simulink library "maggyroProcessing_lib"  (R2018b)
settings: Solver=VariableStepAuto  StartTime=0.0  StopTime=10.0  RelTol=1e-3
undefined symbols (not defined in the file or in its folder): fswParams, u1, unit_conversion
libraries: dspindex x18, two_norm x9, simulink x7
settings Model: Creator=sophiakim  LastModifiedBy=Taylor

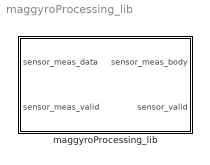
== system maggyroProcessing_lib ==
  maggyroProcessing_lib : Subsystem  TreatAsAtomicUnit=on  mask{static_range_max_value=fswParams.sensors.gyro_static_range, offset_calibration_matrix=fswParams.sensors.gyro_offset, max_err=fswParams.sensors.mag_max_err, rotation_calibration_matrix=fswParams.sensors.gyro_rotate, Gain=unit_conversion}
      mask prompts: static_range_max_value "Max Static Range"; offset_calibration_matrix "Offset Calibration Matrix"; max_err "Max Error Between Signals Allowed"; rotation_calibration_matrix "3x3x3 Matrix of Rotation Matrices"; Gain "Measurement-to-FSW Unit Conversion"
      settings: RTWFcnNameOpts=Use subsystem name  RTWFileNameOpts=Use subsystem name
      mask TypeOptions static_range_max_value:
      | StaticRangeCheck
      | /Check
      | Static Range1/max | StaticRangeCheck
      | /Check
      | Static Range2/max | StaticRangeCheck
      | /Check
      | Static Range4/max
      mask TypeOptions offset_calibration_matrix: DataCalibration/mag_offset/Value
      mask TypeOptions Gain: UnitConversion/Gain
      mask DialogControl DescTextVar Prompt: Provide the sensor (mag or gyro) measurements in the sensor frame(s), as well as the individual validity flags. This library then blends the three measurements into a single three-dimensional vector and a single validity flag.

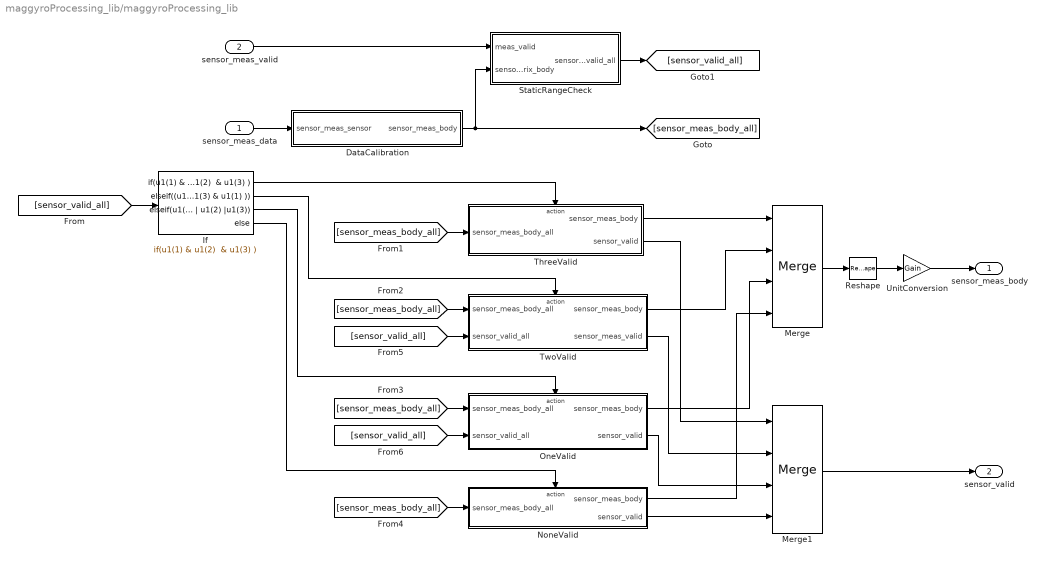
== system maggyroProcessing_lib/maggyroProcessing_lib ==
  sensor_meas_data : Inport
  sensor_meas_valid : Inport  Port=2
  DataCalibration : Subsystem
  If : If  IfExpression="u1(1) & u1(2)  & u1(3)"  ElseIfExpressions=(u1(1) & u1(2) ) | (u1(2) & u1(3) )|(u1(3) & u1(1) ), u1(1) | u1(2) |u1(3)
  Merge : Merge  Inputs=4
  Merge1 : Merge  Inputs=4
  NoneValid : Subsystem  TreatAsAtomicUnit=on
  OneValid : Subsystem  TreatAsAtomicUnit=on
  Reshape : Reshape
  "StaticRangeCheck " : Subsystem
  ThreeValid : Subsystem  TreatAsAtomicUnit=on
  TwoValid : Subsystem  TreatAsAtomicUnit=on
  UnitConversion : Gain  Gain=Gain
  sensor_meas_body : Outport
  sensor_valid : Outport  Port=2
  wires:
  "StaticRangeCheck "/1(sensor_valid_all) -> [sensor_valid_all]
  NoneValid/2(sensor_valid) -> Merge1/4
  If/4 -> NoneValid/Action
  [sensor_valid_all] -> If/1
  [sensor_meas_body_all] -> OneValid/1(sensor_meas_body_all)
  [sensor_valid_all] -> OneValid/2(sensor_valid_all)
  OneValid/1(sensor_meas_body) -> Merge/3
  TwoValid/2(sensor_meas_valid) -> Merge1/2
  NoneValid/1(sensor_meas_body) -> Merge/4
  [sensor_meas_body_all] -> TwoValid/1(sensor_meas_body_all)
  If/1 -> ThreeValid/Action
  If/2 -> TwoValid/Action
  If/3 -> OneValid/Action
  OneValid/2(sensor_valid) -> Merge1/3
  TwoValid/1(sensor_meas_body) -> Merge/2
  [sensor_meas_body_all] -> NoneValid/1(sensor_meas_body_all)
  [sensor_valid_all] -> TwoValid/2(sensor_valid_all)
  Merge/1 -> Reshape/1
  Merge1/1 -> sensor_valid/1
  sensor_meas_valid/1 -> "StaticRangeCheck "/1(meas_valid)
  sensor_meas_data/1 -> DataCalibration/1(sensor_meas_sensor)
  DataCalibration/1(sensor_meas_body) -> "StaticRangeCheck "/2(sensor_matrix_body), [sensor_meas_body_all]
  ThreeValid/1(sensor_meas_body) -> Merge/1
  ThreeValid/2(sensor_valid) -> Merge1/1
  [sensor_meas_body_all] -> ThreeValid/1(sensor_meas_body_all)
  Reshape/1 -> UnitConversion/1
  UnitConversion/1 -> sensor_meas_body/1

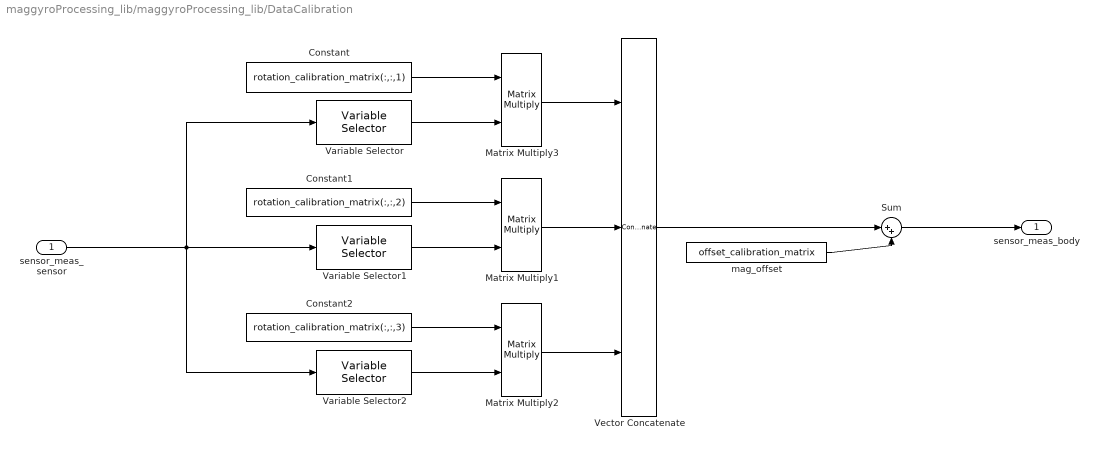
== system maggyroProcessing_lib/maggyroProcessing_lib/DataCalibration ==
  sensor_meas_sensor : Inport
  Constant : Constant  Value=rotation_calibration_matrix(:,:,1)
  Constant1 : Constant  Value=rotation_calibration_matrix(:,:,2)
  Constant2 : Constant  Value=rotation_calibration_matrix(:,:,3)
  Matrix Multiply1 : Product  Multiplication=Matrix(*)
  Matrix Multiply2 : Product  Multiplication=Matrix(*)
  Matrix Multiply3 : Product  Multiplication=Matrix(*)
  Sum : Sum  Inputs=|++
  Variable Selector : dspindex/Variable Selector  NumInputs=1  rowsOrCols=Columns  IdxMode=Fixed  Elements=[1]  ZerOneIdxMode=One-based  errmode=Clip Index  FillMode=on  FillValues=0
  Variable Selector1 : dspindex/Variable Selector  NumInputs=1  rowsOrCols=Columns  IdxMode=Fixed  Elements=[2]  ZerOneIdxMode=One-based  errmode=Clip Index  FillMode=on  FillValues=0
  Variable Selector2 : dspindex/Variable Selector  NumInputs=1  rowsOrCols=Columns  IdxMode=Fixed  Elements=[3]  ZerOneIdxMode=One-based  errmode=Clip Index  FillMode=on  FillValues=0
  Vector Concatenate : Concatenate  NumInputs=3  Mode=Multidimensional array  ConcatenateDimension=2
  mag_offset : Constant  Value=offset_calibration_matrix
  sensor_meas_body : Outport
  wires:
  mag_offset/1 -> Sum/2
  Sum/1 -> sensor_meas_body/1
  sensor_meas_sensor/1 -> Variable Selector/1, Variable Selector2/1, Variable Selector1/1
  Variable Selector/1 -> Matrix Multiply3/2
  Constant/1 -> Matrix Multiply3/1
  Variable Selector1/1 -> Matrix Multiply1/2
  Variable Selector2/1 -> Matrix Multiply2/2
  Constant1/1 -> Matrix Multiply1/1
  Constant2/1 -> Matrix Multiply2/1
  Matrix Multiply3/1 -> Vector Concatenate/1
  Matrix Multiply1/1 -> Vector Concatenate/2
  Matrix Multiply2/1 -> Vector Concatenate/3
  Vector Concatenate/1 -> Sum/1

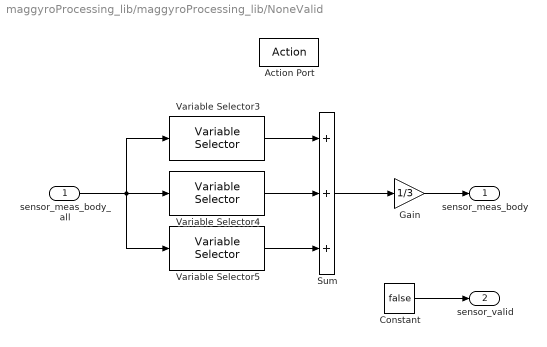
== system maggyroProcessing_lib/maggyroProcessing_lib/NoneValid ==
  sensor_meas_body_all : Inport
  Action Port : ActionPort
  Constant : Constant  Value=false
  Gain : Gain  Gain=1/3
  Sum : Sum  Inputs=+++
  Variable Selector3 : dspindex/Variable Selector  NumInputs=1  rowsOrCols=Columns  IdxMode=Fixed  Elements=[1]  ZerOneIdxMode=One-based  errmode=Clip Index  FillMode=on  FillValues=0
  Variable Selector4 : dspindex/Variable Selector  NumInputs=1  rowsOrCols=Columns  IdxMode=Fixed  Elements=[2]  ZerOneIdxMode=One-based  errmode=Clip Index  FillMode=on  FillValues=0
  Variable Selector5 : dspindex/Variable Selector  NumInputs=1  rowsOrCols=Columns  IdxMode=Fixed  Elements=[3]  ZerOneIdxMode=One-based  errmode=Clip Index  FillMode=on  FillValues=0
  sensor_meas_body : Outport
  sensor_valid : Outport  Port=2
  wires:
  Sum/1 -> Gain/1
  Variable Selector5/1 -> Sum/3
  Variable Selector4/1 -> Sum/2
  Variable Selector3/1 -> Sum/1
  sensor_meas_body_all/1 -> Variable Selector5/1, Variable Selector3/1, Variable Selector4/1
  Gain/1 -> sensor_meas_body/1
  Constant/1 -> sensor_valid/1

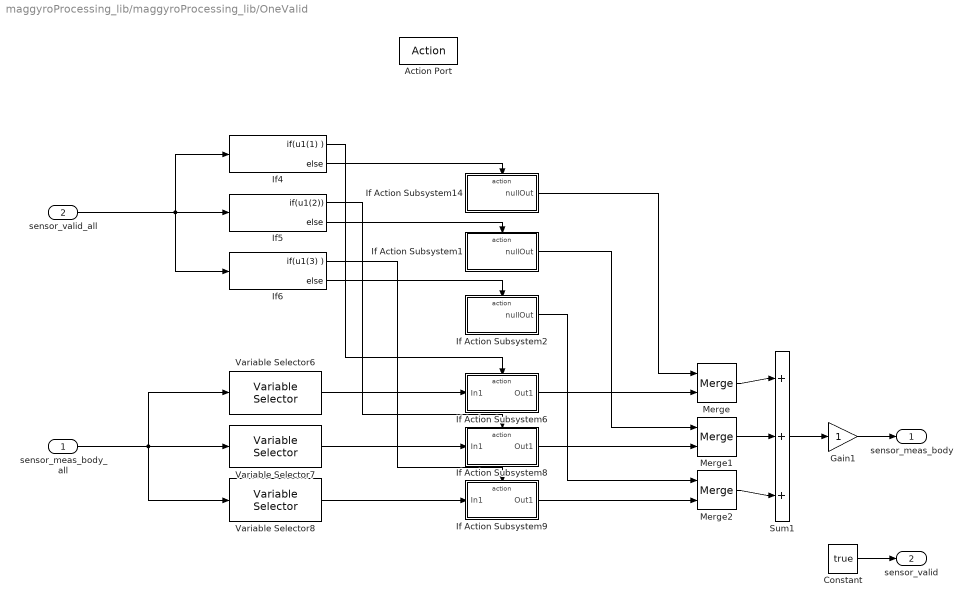
== system maggyroProcessing_lib/maggyroProcessing_lib/OneValid ==
  sensor_meas_body_all : Inport
  sensor_valid_all : Inport  Port=2
  Action Port : ActionPort
  Constant : Constant  Value=true
  Gain1 : Gain
  If Action Subsystem1 : Subsystem  TreatAsAtomicUnit=on
  If Action Subsystem14 : Subsystem  TreatAsAtomicUnit=on
  If Action Subsystem2 : Subsystem  TreatAsAtomicUnit=on
  If Action Subsystem6 : Subsystem  TreatAsAtomicUnit=on
  If Action Subsystem8 : Subsystem  TreatAsAtomicUnit=on
  If Action Subsystem9 : Subsystem  TreatAsAtomicUnit=on
  If4 : If  IfExpression=u1(1)
  If5 : If  IfExpression=u1(2)
  If6 : If  IfExpression=u1(3)
  Merge : Merge
  Merge1 : Merge
  Merge2 : Merge
  Sum1 : Sum  Inputs=+++
  Variable Selector6 : dspindex/Variable Selector  NumInputs=1  rowsOrCols=Columns  IdxMode=Fixed  Elements=[1]  ZerOneIdxMode=One-based  errmode=Clip Index  FillMode=on  FillValues=0
  Variable Selector7 : dspindex/Variable Selector  NumInputs=1  rowsOrCols=Columns  IdxMode=Fixed  Elements=[2]  ZerOneIdxMode=One-based  errmode=Clip Index  FillMode=on  FillValues=0
  Variable Selector8 : dspindex/Variable Selector  NumInputs=1  rowsOrCols=Columns  IdxMode=Fixed  Elements=[3]  ZerOneIdxMode=One-based  errmode=Clip Index  FillMode=on  FillValues=0
  sensor_meas_body : Outport
  sensor_valid : Outport  Port=2
  wires:
  Gain1/1 -> sensor_meas_body/1
  If Action Subsystem6/1(Out1) -> Merge/2
  If4/2 -> If Action Subsystem14/Action
  If6/1 -> If Action Subsystem9/Action
  Sum1/1 -> Gain1/1
  If4/1 -> If Action Subsystem6/Action
  Variable Selector8/1 -> If Action Subsystem9/1(In1)
  Variable Selector6/1 -> If Action Subsystem6/1(In1)
  If Action Subsystem1/1(nullOut) -> Merge1/1
  If5/1 -> If Action Subsystem8/Action
  Merge/1 -> Sum1/1
  If Action Subsystem9/1(Out1) -> Merge2/2
  If Action Subsystem2/1(nullOut) -> Merge2/1
  Merge2/1 -> Sum1/3
  If Action Subsystem8/1(Out1) -> Merge1/2
  Variable Selector7/1 -> If Action Subsystem8/1(In1)
  Merge1/1 -> Sum1/2
  If6/2 -> If Action Subsystem2/Action
  If Action Subsystem14/1(nullOut) -> Merge/1
  If5/2 -> If Action Subsystem1/Action
  sensor_meas_body_all/1 -> Variable Selector6/1, Variable Selector8/1, Variable Selector7/1
  sensor_valid_all/1 -> If6/1, If4/1, If5/1
  Constant/1 -> sensor_valid/1

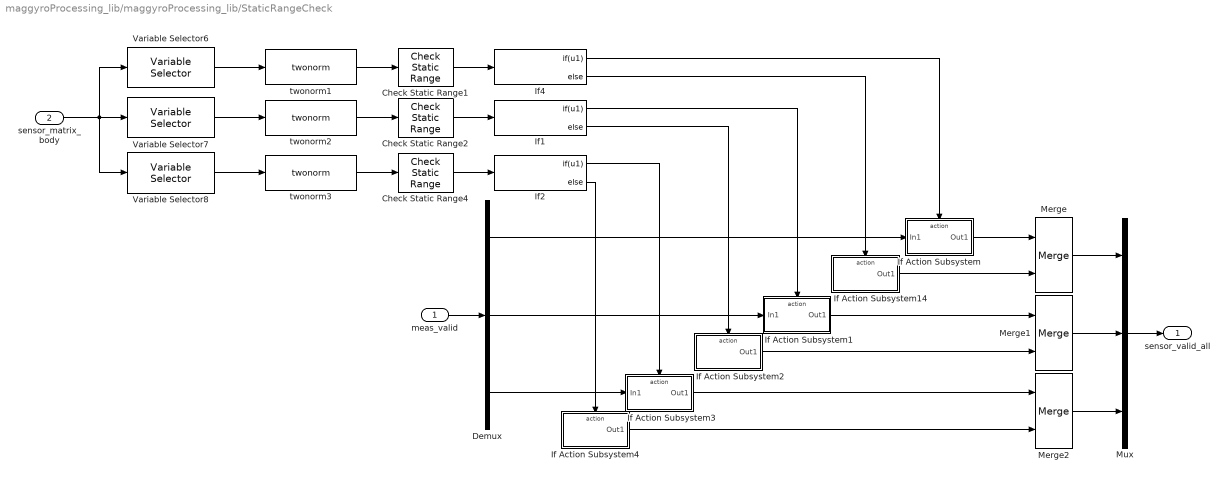
== system maggyroProcessing_lib/maggyroProcessing_lib/StaticRangeCheck  ==
  meas_valid : Inport
  sensor_matrix_body : Inport  Port=2
  Check Static Range1 : simulink/Model Verification/Check  Static Range  Description=0 <= u <= static_range_max_value  max=static_range_max_value  max_included=on  min=0  min_included=on  enabled=on  stopWhenAssertionFail=off  export=on  icon=graphic
      settings: SourceProductName=Simulink  SourceProductBaseCode=SL
  Check Static Range2 : simulink/Model Verification/Check  Static Range  Description=0 <= u <= static_range_max_value  max=static_range_max_value  max_included=on  min=0  min_included=on  enabled=on  stopWhenAssertionFail=off  export=on  icon=graphic
      settings: SourceProductName=Simulink  SourceProductBaseCode=SL
  Check Static Range4 : simulink/Model Verification/Check  Static Range  Description=0 <= u <= static_range_max_value  max=static_range_max_value  max_included=on  min=0  min_included=on  enabled=on  stopWhenAssertionFail=off  export=on  icon=graphic
      settings: SourceProductName=Simulink  SourceProductBaseCode=SL
  Demux : Demux  Outputs=3
  If Action Subsystem : Subsystem  TreatAsAtomicUnit=on
  If Action Subsystem1 : Subsystem  TreatAsAtomicUnit=on
  If Action Subsystem14 : Subsystem  TreatAsAtomicUnit=on
  If Action Subsystem2 : Subsystem  TreatAsAtomicUnit=on
  If Action Subsystem3 : Subsystem  TreatAsAtomicUnit=on
  If Action Subsystem4 : Subsystem  TreatAsAtomicUnit=on
  If1 : If  IfExpression=u1
  If2 : If  IfExpression=u1
  If4 : If  IfExpression=u1
  Merge : Merge
  Merge1 : Merge
  Merge2 : Merge
  Mux : Mux  Inputs=3
  Variable Selector6 : dspindex/Variable Selector  NumInputs=1  rowsOrCols=Columns  IdxMode=Fixed  Elements=[1]  ZerOneIdxMode=One-based  errmode=Clip Index  FillMode=on  FillValues=0
  Variable Selector7 : dspindex/Variable Selector  NumInputs=1  rowsOrCols=Columns  IdxMode=Fixed  Elements=[2]  ZerOneIdxMode=One-based  errmode=Clip Index  FillMode=on  FillValues=0
  Variable Selector8 : dspindex/Variable Selector  NumInputs=1  rowsOrCols=Columns  IdxMode=Fixed  Elements=[3]  ZerOneIdxMode=One-based  errmode=Clip Index  FillMode=on  FillValues=0
  twonorm1 : two_norm/twonorm  SystemSampleTime=-1
  twonorm2 : two_norm/twonorm  SystemSampleTime=-1
  twonorm3 : two_norm/twonorm  SystemSampleTime=-1
  sensor_valid_all : Outport
  wires:
  If2/2 -> If Action Subsystem4/Action
  If2/1 -> If Action Subsystem3/Action
  If4/2 -> If Action Subsystem14/Action
  Check Static Range1/1 -> If4/1
  If4/1 -> If Action Subsystem/Action
  Check Static Range4/1 -> If2/1
  If1/2 -> If Action Subsystem2/Action
  Demux/1 -> If Action Subsystem/1(In1)
  If1/1 -> If Action Subsystem1/Action
  If Action Subsystem/1(Out1) -> Merge/1
  If Action Subsystem14/1(Out1) -> Merge/2
  If Action Subsystem1/1(Out1) -> Merge1/1
  If Action Subsystem2/1(Out1) -> Merge1/2
  If Action Subsystem3/1(Out1) -> Merge2/1
  If Action Subsystem4/1(Out1) -> Merge2/2
  Demux/3 -> If Action Subsystem3/1(In1)
  Merge/1 -> Mux/1
  Merge1/1 -> Mux/2
  Merge2/1 -> Mux/3
  Mux/1 -> sensor_valid_all/1
  sensor_matrix_body/1 -> Variable Selector8/1, Variable Selector7/1, Variable Selector6/1
  Check Static Range2/1 -> If1/1
  Variable Selector6/1 -> twonorm1/1
  Variable Selector7/1 -> twonorm2/1
  Variable Selector8/1 -> twonorm3/1
  meas_valid/1 -> Demux/1
  Demux/2 -> If Action Subsystem1/1(In1)
  twonorm1/1 -> Check Static Range1/1
  twonorm2/1 -> Check Static Range2/1
  twonorm3/1 -> Check Static Range4/1

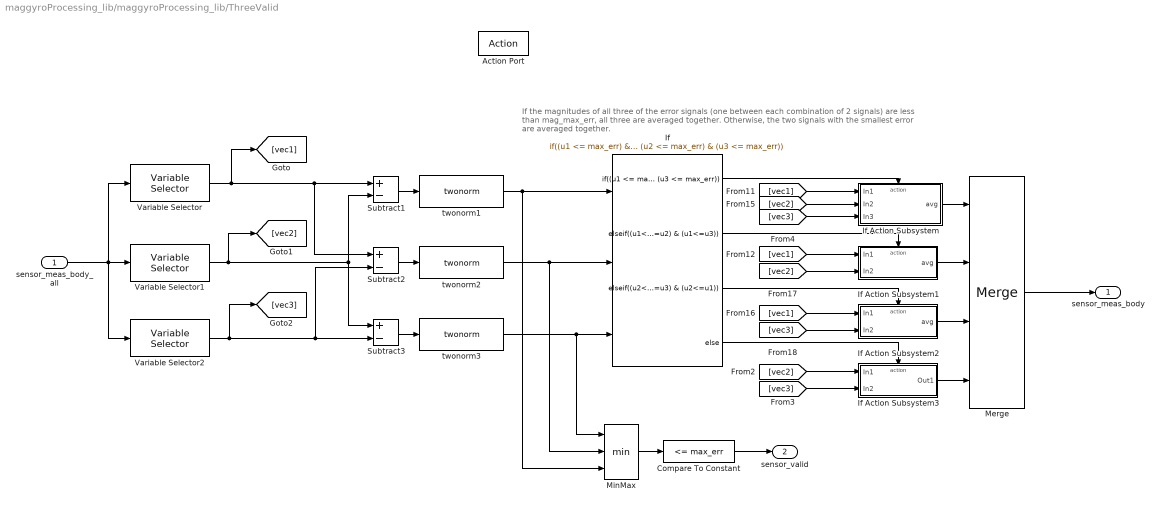
== system maggyroProcessing_lib/maggyroProcessing_lib/ThreeValid ==
  note: If the magnitudes of all three of the error signals (one between each combination of 2 signals)
      | are less than mag_max_err, all three are averaged together. Otherwise, the two signals with the
      | smallest error are averaged together.
  sensor_meas_body_all : Inport
  Action Port : ActionPort
  Compare To Constant : simulink/Logic and Bit Operations/Compare To Constant  relop=<=  const=max_err  OutDataTypeStr=boolean
  If : If  NumInputs=3  IfExpression=(u1 <= max_err) & (u2 <= max_err) & (u3 <= max_err)  ElseIfExpressions=(u1<=u2) & (u1<=u3),(u2<=u3) & (u2<=u1)
  If Action Subsystem : Subsystem  TreatAsAtomicUnit=on
  If Action Subsystem1 : Subsystem  TreatAsAtomicUnit=on
  If Action Subsystem2 : Subsystem  TreatAsAtomicUnit=on
  If Action Subsystem3 : Subsystem  TreatAsAtomicUnit=on
  Merge : Merge  Inputs=4
  MinMax : MinMax  Inputs=3
  Subtract1 : Sum  Inputs=+-
  Subtract2 : Sum  Inputs=+-
  Subtract3 : Sum  Inputs=+-
  Variable Selector : dspindex/Variable Selector  NumInputs=1  rowsOrCols=Columns  IdxMode=Fixed  Elements=[1]  ZerOneIdxMode=One-based  errmode=Clip Index  FillMode=on  FillValues=0
  Variable Selector1 : dspindex/Variable Selector  NumInputs=1  rowsOrCols=Columns  IdxMode=Fixed  Elements=[2]  ZerOneIdxMode=One-based  errmode=Clip Index  FillMode=on  FillValues=0
  Variable Selector2 : dspindex/Variable Selector  NumInputs=1  rowsOrCols=Columns  IdxMode=Fixed  Elements=[3]  ZerOneIdxMode=One-based  errmode=Clip Index  FillMode=on  FillValues=0
  twonorm1 : two_norm/twonorm  SystemSampleTime=-1
  twonorm2 : two_norm/twonorm  SystemSampleTime=-1
  twonorm3 : two_norm/twonorm  SystemSampleTime=-1
  sensor_meas_body : Outport
  sensor_valid : Outport  Port=2
  wires:
  twonorm3/1 -> MinMax/1, If/3
  twonorm2/1 -> MinMax/2, If/2
  twonorm1/1 -> MinMax/3, If/1
  Variable Selector/1 -> Subtract2/1, Subtract1/1, [vec1]
  Subtract1/1 -> twonorm1/1
  Subtract3/1 -> twonorm3/1
  [vec1] -> If Action Subsystem/1(In1)
  [vec1] -> If Action Subsystem1/1(In1)
  [vec2] -> If Action Subsystem/2(In2)
  [vec2] -> If Action Subsystem1/2(In2)
  Variable Selector1/1 -> Subtract1/2, Subtract3/1, [vec2]
  If/2 -> If Action Subsystem1/Action
  Variable Selector2/1 -> Subtract2/2, Subtract3/2, [vec3]
  If/3 -> If Action Subsystem2/Action
  Subtract2/1 -> twonorm2/1
  If/1 -> If Action Subsystem/Action
  If Action Subsystem/1(avg) -> Merge/1
  sensor_meas_body_all/1 -> Variable Selector/1, Variable Selector1/1, Variable Selector2/1
  If Action Subsystem1/1(avg) -> Merge/2
  If Action Subsystem2/1(avg) -> Merge/3
  Merge/1 -> sensor_meas_body/1
  MinMax/1 -> Compare To Constant/1
  Compare To Constant/1 -> sensor_valid/1
  [vec3] -> If Action Subsystem/3(In3)
  If/4 -> If Action Subsystem3/Action
  [vec3] -> If Action Subsystem2/2(In2)
  [vec1] -> If Action Subsystem2/1(In1)
  If Action Subsystem3/1(Out1) -> Merge/4
  [vec2] -> If Action Subsystem3/1(In1)
  [vec3] -> If Action Subsystem3/2(In2)

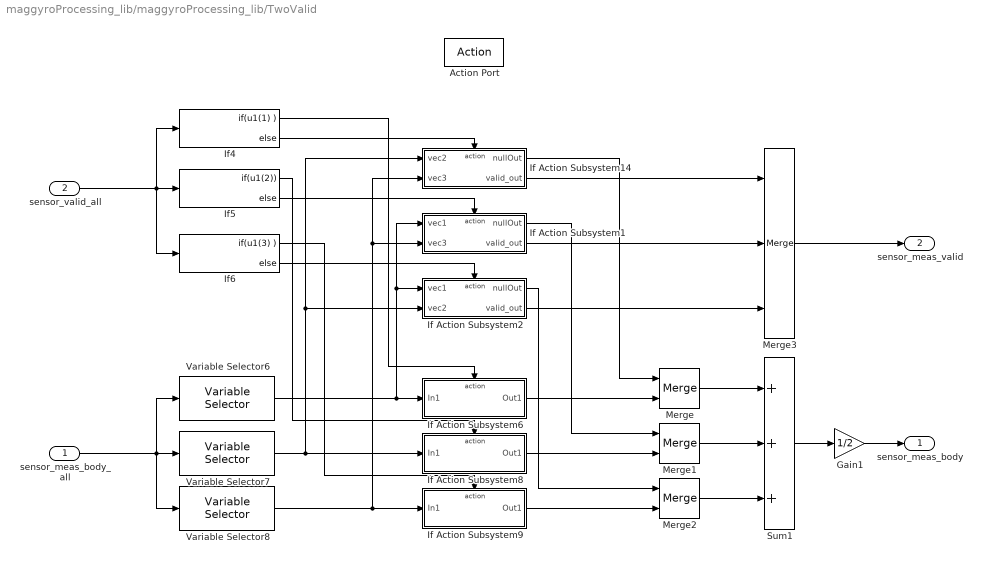
== system maggyroProcessing_lib/maggyroProcessing_lib/TwoValid ==
  sensor_meas_body_all : Inport
  sensor_valid_all : Inport  Port=2
  Action Port : ActionPort
  Gain1 : Gain  Gain=1/2
  If Action Subsystem1 : Subsystem  TreatAsAtomicUnit=on
  If Action Subsystem14 : Subsystem  TreatAsAtomicUnit=on
  If Action Subsystem2 : Subsystem  TreatAsAtomicUnit=on
  If Action Subsystem6 : Subsystem  TreatAsAtomicUnit=on
  If Action Subsystem8 : Subsystem  TreatAsAtomicUnit=on
  If Action Subsystem9 : Subsystem  TreatAsAtomicUnit=on
  If4 : If  IfExpression=u1(1)
  If5 : If  IfExpression=u1(2)
  If6 : If  IfExpression=u1(3)
  Merge : Merge
  Merge1 : Merge
  Merge2 : Merge
  Merge3 : Merge  Inputs=3
  Sum1 : Sum  Inputs=+++
  Variable Selector6 : dspindex/Variable Selector  NumInputs=1  rowsOrCols=Columns  IdxMode=Fixed  Elements=[1]  ZerOneIdxMode=One-based  errmode=Clip Index  FillMode=on  FillValues=0
  Variable Selector7 : dspindex/Variable Selector  NumInputs=1  rowsOrCols=Columns  IdxMode=Fixed  Elements=[2]  ZerOneIdxMode=One-based  errmode=Clip Index  FillMode=on  FillValues=0
  Variable Selector8 : dspindex/Variable Selector  NumInputs=1  rowsOrCols=Columns  IdxMode=Fixed  Elements=[3]  ZerOneIdxMode=One-based  errmode=Clip Index  FillMode=on  FillValues=0
  sensor_meas_body : Outport
  sensor_meas_valid : Outport  Port=2
  wires:
  Variable Selector7/1 -> If Action Subsystem2/2(vec2), If Action Subsystem14/1(vec2), If Action Subsystem8/1(In1)
  sensor_valid_all/1 -> If6/1, If4/1, If5/1
  If5/1 -> If Action Subsystem8/Action
  If6/1 -> If Action Subsystem9/Action
  If4/1 -> If Action Subsystem6/Action
  Variable Selector6/1 -> If Action Subsystem2/1(vec1), If Action Subsystem1/1(vec1), If Action Subsystem6/1(In1)
  Variable Selector8/1 -> If Action Subsystem1/2(vec3), If Action Subsystem14/2(vec3), If Action Subsystem9/1(In1)
  Gain1/1 -> sensor_meas_body/1
  Sum1/1 -> Gain1/1
  sensor_meas_body_all/1 -> Variable Selector8/1, Variable Selector7/1, Variable Selector6/1
  If4/2 -> If Action Subsystem14/Action
  If Action Subsystem14/1(nullOut) -> Merge/1
  If Action Subsystem6/1(Out1) -> Merge/2
  Merge/1 -> Sum1/1
  If Action Subsystem8/1(Out1) -> Merge1/2
  If Action Subsystem9/1(Out1) -> Merge2/2
  Merge2/1 -> Sum1/3
  Merge1/1 -> Sum1/2
  If5/2 -> If Action Subsystem1/Action
  If6/2 -> If Action Subsystem2/Action
  If Action Subsystem1/1(nullOut) -> Merge1/1
  If Action Subsystem2/1(nullOut) -> Merge2/1
  If Action Subsystem14/2(valid_out) -> Merge3/1
  If Action Subsystem1/2(valid_out) -> Merge3/2
  If Action Subsystem2/2(valid_out) -> Merge3/3
  Merge3/1 -> sensor_meas_valid/1

== system maggyroProcessing_lib/maggyroProcessing_lib/OneValid/If Action Subsystem1 ==
  Action Port : ActionPort
  Constant : Constant  Value=[0;0;0]
  nullOut : Outport
  wires:
  Constant/1 -> nullOut/1

== system maggyroProcessing_lib/maggyroProcessing_lib/OneValid/If Action Subsystem14 ==
  Action Port : ActionPort
  Constant : Constant  Value=[0;0;0]
  nullOut : Outport
  wires:
  Constant/1 -> nullOut/1

== system maggyroProcessing_lib/maggyroProcessing_lib/OneValid/If Action Subsystem2 ==
  Action Port : ActionPort
  Constant : Constant  Value=[0;0;0]
  nullOut : Outport
  wires:
  Constant/1 -> nullOut/1

== system maggyroProcessing_lib/maggyroProcessing_lib/OneValid/If Action Subsystem6 ==
  In1 : Inport
  Action Port : ActionPort
  Out1 : Outport
  wires:
  In1/1 -> Out1/1

== system maggyroProcessing_lib/maggyroProcessing_lib/OneValid/If Action Subsystem8 ==
  In1 : Inport
  Action Port : ActionPort
  Out1 : Outport
  wires:
  In1/1 -> Out1/1

== system maggyroProcessing_lib/maggyroProcessing_lib/OneValid/If Action Subsystem9 ==
  In1 : Inport
  Action Port : ActionPort
  Out1 : Outport
  wires:
  In1/1 -> Out1/1

== system maggyroProcessing_lib/maggyroProcessing_lib/StaticRangeCheck /If Action Subsystem ==
  In1 : Inport
  Action Port : ActionPort
  Out1 : Outport
  wires:
  In1/1 -> Out1/1

== system maggyroProcessing_lib/maggyroProcessing_lib/StaticRangeCheck /If Action Subsystem1 ==
  In1 : Inport
  Action Port : ActionPort
  Out1 : Outport
  wires:
  In1/1 -> Out1/1

== system maggyroProcessing_lib/maggyroProcessing_lib/StaticRangeCheck /If Action Subsystem14 ==
  Action Port : ActionPort
  Constant : Constant  Value=0  OutDataTypeStr=boolean
  Out1 : Outport
  wires:
  Constant/1 -> Out1/1

== system maggyroProcessing_lib/maggyroProcessing_lib/StaticRangeCheck /If Action Subsystem2 ==
  Action Port : ActionPort
  Constant : Constant  Value=0  OutDataTypeStr=boolean
  Out1 : Outport
  wires:
  Constant/1 -> Out1/1

== system maggyroProcessing_lib/maggyroProcessing_lib/StaticRangeCheck /If Action Subsystem3 ==
  In1 : Inport
  Action Port : ActionPort
  Out1 : Outport
  wires:
  In1/1 -> Out1/1

== system maggyroProcessing_lib/maggyroProcessing_lib/StaticRangeCheck /If Action Subsystem4 ==
  Action Port : ActionPort
  Constant : Constant  Value=0  OutDataTypeStr=boolean
  Out1 : Outport
  wires:
  Constant/1 -> Out1/1

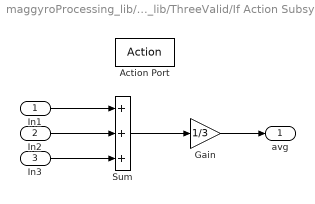
== system maggyroProcessing_lib/maggyroProcessing_lib/ThreeValid/If Action Subsystem ==
  In1 : Inport
  In2 : Inport  Port=2
  In3 : Inport  Port=3
  Action Port : ActionPort
  Gain : Gain  Gain=1/3
  Sum : Sum  Inputs=+++
  avg : Outport
  wires:
  In1/1 -> Sum/1
  In2/1 -> Sum/2
  Sum/1 -> Gain/1
  Gain/1 -> avg/1
  In3/1 -> Sum/3

== system maggyroProcessing_lib/maggyroProcessing_lib/ThreeValid/If Action Subsystem1 ==
  In1 : Inport
  In2 : Inport  Port=2
  Action Port : ActionPort  ActionType=elseif
  Gain : Gain  Gain=1/2
  Sum : Sum
  avg : Outport
  wires:
  In2/1 -> Sum/2
  In1/1 -> Sum/1
  Gain/1 -> avg/1
  Sum/1 -> Gain/1

== system maggyroProcessing_lib/maggyroProcessing_lib/ThreeValid/If Action Subsystem2 ==
  In1 : Inport
  In2 : Inport  Port=2
  Action Port : ActionPort  ActionType=elseif
  Gain : Gain  Gain=1/2
  Sum : Sum
  avg : Outport
  wires:
  Sum/1 -> Gain/1
  Gain/1 -> avg/1
  In1/1 -> Sum/1
  In2/1 -> Sum/2

== system maggyroProcessing_lib/maggyroProcessing_lib/ThreeValid/If Action Subsystem3 ==
  In1 : Inport
  In2 : Inport  Port=2
  Action Port : ActionPort  ActionType=else
  Gain : Gain  Gain=1/2
  Sum : Sum
  Out1 : Outport
  wires:
  Sum/1 -> Gain/1
  Gain/1 -> Out1/1
  In1/1 -> Sum/1
  In2/1 -> Sum/2

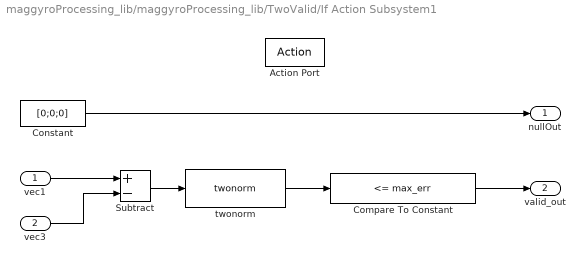
== system maggyroProcessing_lib/maggyroProcessing_lib/TwoValid/If Action Subsystem1 ==
  vec1 : Inport
  vec3 : Inport  Port=2
  Action Port : ActionPort
  Compare To Constant : simulink/Logic and Bit Operations/Compare To Constant  relop=<=  const=max_err  OutDataTypeStr=boolean
  Constant : Constant  Value=[0;0;0]
  Subtract : Sum  Inputs=+-
  twonorm : two_norm/twonorm  SystemSampleTime=-1
  nullOut : Outport
  valid_out : Outport  Port=2
  wires:
  Constant/1 -> nullOut/1
  Subtract/1 -> twonorm/1
  vec1/1 -> Subtract/1
  vec3/1 -> Subtract/2
  Compare To Constant/1 -> valid_out/1
  twonorm/1 -> Compare To Constant/1

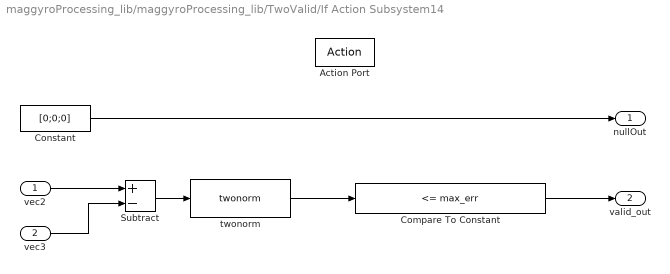
== system maggyroProcessing_lib/maggyroProcessing_lib/TwoValid/If Action Subsystem14 ==
  vec2 : Inport
  vec3 : Inport  Port=2
  Action Port : ActionPort
  Compare To Constant : simulink/Logic and Bit Operations/Compare To Constant  relop=<=  const=max_err  OutDataTypeStr=boolean
  Constant : Constant  Value=[0;0;0]
  Subtract : Sum  Inputs=+-
  twonorm : two_norm/twonorm  SystemSampleTime=-1
  nullOut : Outport
  valid_out : Outport  Port=2
  wires:
  Constant/1 -> nullOut/1
  vec2/1 -> Subtract/1
  vec3/1 -> Subtract/2
  Subtract/1 -> twonorm/1
  Compare To Constant/1 -> valid_out/1
  twonorm/1 -> Compare To Constant/1

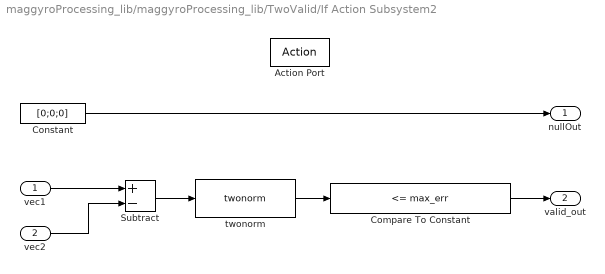
== system maggyroProcessing_lib/maggyroProcessing_lib/TwoValid/If Action Subsystem2 ==
  vec1 : Inport
  vec2 : Inport  Port=2
  Action Port : ActionPort
  Compare To Constant : simulink/Logic and Bit Operations/Compare To Constant  relop=<=  const=max_err  OutDataTypeStr=boolean
  Constant : Constant  Value=[0;0;0]
  Subtract : Sum  Inputs=+-
  twonorm : two_norm/twonorm  SystemSampleTime=-1
  nullOut : Outport
  valid_out : Outport  Port=2
  wires:
  Constant/1 -> nullOut/1
  Subtract/1 -> twonorm/1
  vec1/1 -> Subtract/1
  vec2/1 -> Subtract/2
  Compare To Constant/1 -> valid_out/1
  twonorm/1 -> Compare To Constant/1

== system maggyroProcessing_lib/maggyroProcessing_lib/TwoValid/If Action Subsystem6 ==
  In1 : Inport
  Action Port : ActionPort
  Out1 : Outport
  wires:
  In1/1 -> Out1/1

== system maggyroProcessing_lib/maggyroProcessing_lib/TwoValid/If Action Subsystem8 ==
  In1 : Inport
  Action Port : ActionPort
  Out1 : Outport
  wires:
  In1/1 -> Out1/1

== system maggyroProcessing_lib/maggyroProcessing_lib/TwoValid/If Action Subsystem9 ==
  In1 : Inport
  Action Port : ActionPort
  Out1 : Outport
  wires:
  In1/1 -> Out1/1
